simulink model "Problem1"  (R2020a)
settings: Solver=VariableStepAuto  StartTime=0.0  StopTime=10.0  RelTol=1e-3
model workspace (MAT data in the model file):
  K1 = 50
  K12 = 100
  M1 = 100
  M2 = 50
  b = 50
settings Model: OrderedModelArguments=off  Creator=tanu  LastModifiedBy=tanu

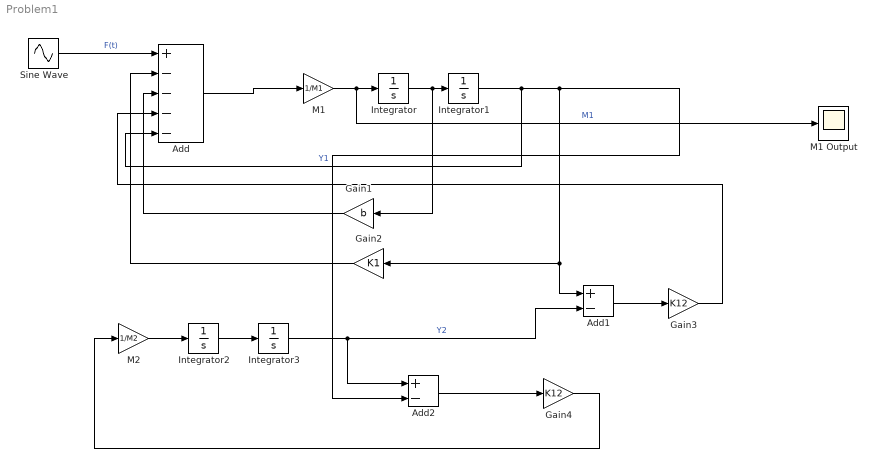
== system Problem1 ==
  Add : Sum  Inputs=+----
  Add1 : Sum  Inputs=+-
  Add2 : Sum  Inputs=+-
  Gain1 : Gain  Gain=b
  Gain2 : Gain  Gain=K1
  Gain3 : Gain  Gain=K12
  Gain4 : Gain  Gain=K12
  Integrator{,1..3} (4 alike) : Integrator
  M1 : Gain  Gain=1/M1
  M1 Output : Scope
  M2 : Gain  Gain=1/M2
  Sine Wave : Sin  Amplitude=2  Frequency=10  SampleTime=0
  wires:
  Sine Wave/1 -> Add/1  "F(t)"
  Add/1 -> M1/1
  M1/1 -> M1 Output/1, Integrator/1  "M1"
  Integrator/1 -> Gain1/1, Integrator1/1
  Integrator1/1 -> Add/5, Add1/1, Gain2/1, Add2/2  "Y1"
  Gain1/1 -> Add/3
  Gain2/1 -> Add/2
  M2/1 -> Integrator2/1
  Integrator2/1 -> Integrator3/1
  Integrator3/1 -> Add2/1, Add1/2  "Y2"
  Gain3/1 -> Add/4
  Add1/1 -> Gain3/1
  Add2/1 -> Gain4/1
  Gain4/1 -> M2/1
